simulink model "sim_part5"  (R2022b)
settings: Solver=VariableStepAuto  StartTime=0.0  StopTime=15  RelTol=1e-3
undefined symbols (not defined in the file): matA1, matB1
libraries: cstblocks x3
settings Model: Creator=alon  LastModifiedBy=binya
settings SolverCC: AlgebraicLoopSolver=TrustRegion
settings DebuggingCC: UnconnectedInputMsg=warning  UnconnectedOutputMsg=warning  UnconnectedLineMsg=warning  SFMachineParentedDataDiag=warning
settings ModelReferenceCC: EnableRefExpFcnMdlSchedulingChecks=on

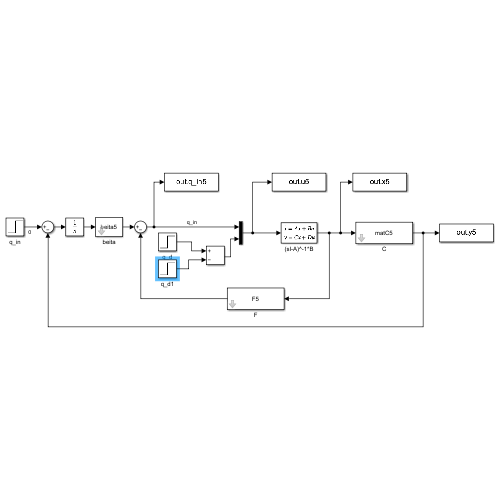
[thumbnail: Simulink's stored preview of the top-level diagram]
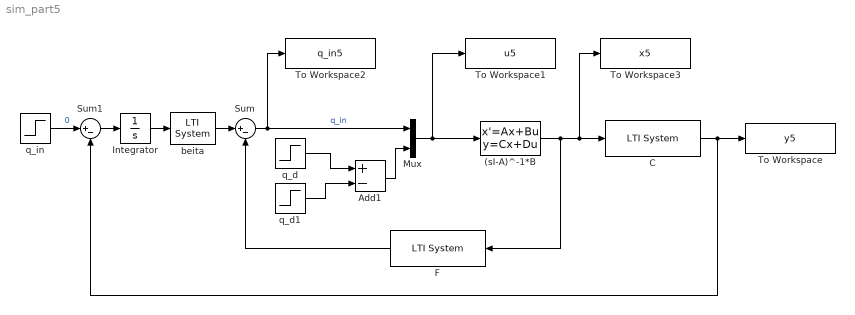
== system sim_part5 ==
  (sI-A)^-1*B : StateSpace  A=matA1  B=matB1  C=eye(3)  D=[[0 0];[0 0];[0 0]]  InitialCondition=0
  Add1 : Sum  Inputs=+-
  C : cstblocks/LTI System  sys=matC5  IC=[]
  F : cstblocks/LTI System  sys=F5  IC=[]
  Integrator : Integrator
  Mux : Mux  Inputs=2
  Sum : Sum  Inputs=|+-
  Sum1 : Sum  Inputs=|+-
  To Workspace : ToWorkspace  VariableName=y5  SaveFormat=Timeseries  SampleTime=-1
  To Workspace1 : ToWorkspace  VariableName=u5  SaveFormat=Timeseries  SampleTime=-1
  To Workspace2 : ToWorkspace  VariableName=q_in5  SaveFormat=Timeseries  SampleTime=-1
  To Workspace3 : ToWorkspace  VariableName=x5  SaveFormat=Timeseries  SampleTime=-1
  beita : cstblocks/LTI System  sys=beita5  IC=[]
  q_d : Step  Time=0  After=12  SampleTime=0
  q_d1 : Step  Time=2.3  After=12  SampleTime=0
  q_in : Step  Time=0  After=0  SampleTime=0
  wires:
  (sI-A)^-1*B/1 -> F/1, To Workspace3/1, C/1
  Sum/1 -> Mux/1, To Workspace2/1  "q_in"
  q_in/1 -> Sum1/1  "0"
  Mux/1 -> To Workspace1/1, (sI-A)^-1*B/1
  q_d1/1 -> Add1/2
  C/1 -> Sum1/2, To Workspace/1
  Add1/1 -> Mux/2
  q_d/1 -> Add1/1
  F/1 -> Sum/2
  Sum1/1 -> Integrator/1
  beita/1 -> Sum/1
  Integrator/1 -> beita/1
